simulink model "Potentiometer_Calibration"  (R2025a)
settings: Solver=ode4  StartTime=0.0  StopTime=inf  FixedStep=0.004  RelTol=1e-3  EnableMultiTasking=on
libraries: raspberrypiCommlib x2
settings Model: SimulationMode=external  ExtModeTrigDuration=2  Creator=Mustafa  LastModifiedBy=chenyihong
settings SolverCC: ExtrapolationOrder=2.0  AlgebraicLoopSolver=TrustRegion  PositivePriorityOrder=on  AutoInsertRateTranBlk=on
settings DataIOCC: ReturnWorkspaceOutputs=off
settings OptimizationCC: PassReuseOutputArgsAs=Individual arguments  MaxStackSize=200000  EfficientTunableParamExpr=on
settings DebuggingCC: ParameterTunabilityLossMsg=error  UnconnectedInputMsg=warning  UnconnectedOutputMsg=warning  UnconnectedLineMsg=warning  ArithmeticOperatorsInVariantConditions=warning
settings HardwareCC: ProdBitPerLong=64.0  ProdLargestAtomicInteger=LongLong  ProdLargestAtomicFloat=Double  ProdLongLongMode=on  ProdHWDeviceType=ARM Compatible->ARM Cortex-A (64-bit)
settings ModelReferenceCC: EnableRefExpFcnMdlSchedulingChecks=on
settings SFSimCC: SimUseLocalCustomCode=off  CustomCodeUndefinedFunction=UseInterfaceOnly
settings RTWCC: SystemTargetFile=ert.tlc  HardwareBoard=Raspberry Pi (64bit)  TLCOptions="-aInlineSetEventsForThisBaseRateFcn=TLC_FALSE -aSuppressMultiTaskScheduler=TLC_FALSE  -aRateBasedStepFcn=0"  TemplateMakefile=ert_default_tmf  GenerateReport=on  RTWUseLocalCustomCode=off  Toolchain=GNU GCC Embedded Linux  BuildConfiguration=Faster Runs  IncludeHyperlinkInReport=on  LaunchReport=on  GenerateTraceInfo=on  GenerateTraceReport=on  GenerateTraceReportSl=on  GenerateTraceReportSf=on  GenerateTraceReportEml=on  GPUComputeCapability=3.5  DLArmComputeVersion=19.05  Description=Embedded Coder
settings CodeAppCC: ForceParamTrailComments=on  IgnoreCustomStorageClasses=off  OperatorAnnotations=on  SimulinkDataObjDesc=on  SFDataObjDesc=on  InsertBlockDesc=on
settings ERTTargetCC: ExtMode=on  ExtModeTransport=2.0  ExtModeMexArgs='127.0.0.1' 0 17725  InlinedParameterPlacement=Hierarchical  DynamicArrayContainerType=coder::array  CodeReplacementLibrary=ARM Cortex-A CMSIS  SupportContinuousTime=on  SupportVariableSizeSignals=on

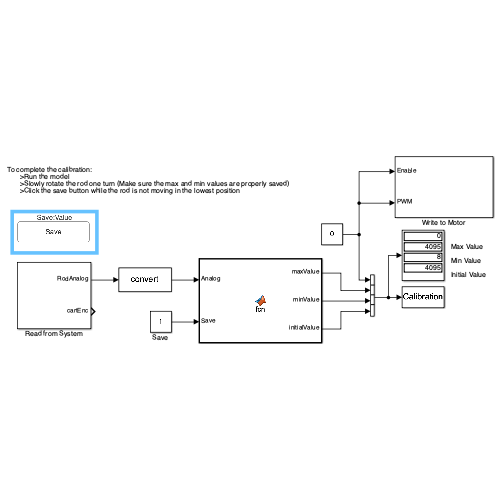
[thumbnail: Simulink's stored preview of the top-level diagram]
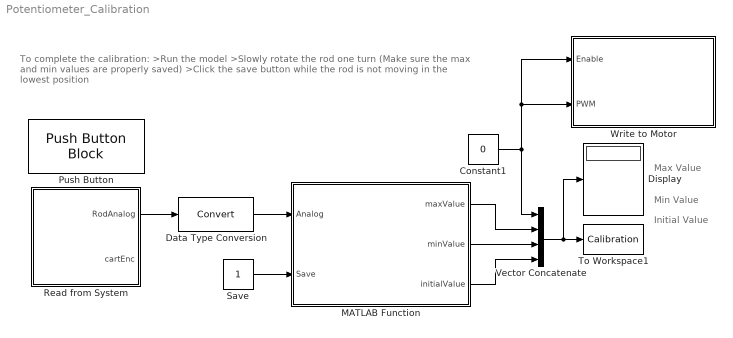
== system Potentiometer_Calibration ==
  note: Min Value
  note: To complete the calibration:
      | >Run the model
      | >Slowly rotate the rod one turn (Make sure the max and min values are properly saved)
      | >Click the save button while the rod is not moving in the lowest position
  note: Initial Value
  note: Max Value
  Constant1 : Constant  Value=0
  Data Type Conversion : DataTypeConversion  SaturateOnIntegerOverflow=off  RndMeth=Floor
  Display : Display
  MATLAB Function : MATLAB Function  TreatAsAtomicUnit=on
  Push Button : PushButtonBlock  LabelPosition=Top  ButtonText=Save  IconOnColor=[0.0, 0.39215686274509803, 0.0]  IconOffColor=[0.0, 1.0, 0.0]  OffValue=1.000000
  Read from System : Subsystem
  Save : Constant
  To Workspace1 : ToWorkspace  VariableName=Calibration  SampleTime=-1
      settings: MaxDataPoints=1
  Vector Concatenate : Concatenate  NumInputs=4
  Write to Motor : Subsystem
  wires:
  MATLAB Function/2(minValue) -> Vector Concatenate/3
  Vector Concatenate/1 -> Display/1, To Workspace1/1
  Constant1/1 -> Vector Concatenate/1, Write to Motor/2(PWM), Write to Motor/1(Enable)
  Save/1 -> MATLAB Function/2(Save)
  Data Type Conversion/1 -> MATLAB Function/1(Analog)
  Read from System/1(RodAnalog) -> Data Type Conversion/1
  MATLAB Function/1(maxValue) -> Vector Concatenate/2
  MATLAB Function/3(initialValue) -> Vector Concatenate/4

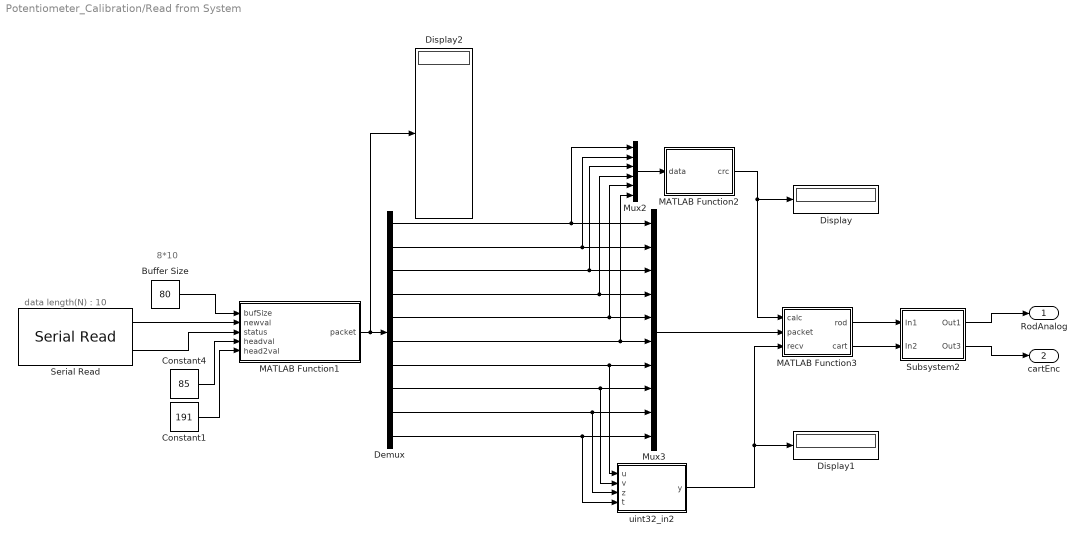
== system Potentiometer_Calibration/Read from System ==
  note: data length(N) : 10
  note: 8*10
  Buffer Size : Constant  Value=80  OutDataTypeStr=uint8
  Constant1 : Constant  Value=191  OutDataTypeStr=uint8
  Constant4 : Constant  Value=85  OutDataTypeStr=uint8
  Demux : Demux  Outputs=10
  Display : Display
  Display1 : Display
  Display2 : Display
  MATLAB Function1 : MATLAB Function  TreatAsAtomicUnit=on
  MATLAB Function2 : MATLAB Function  TreatAsAtomicUnit=on
  MATLAB Function3 : MATLAB Function  TreatAsAtomicUnit=on
  Mux2 : Mux  Inputs=6
  Mux3 : Mux  Inputs=10
  Serial Read : raspberrypiCommlib/Serial Read  board=Pi 3 Model B  SCIModule_=/dev/serial0  Baudrate_=115200  Parity=None  StopBits_=1  HardwareFlowControl=None  ByteOrder=LittleEndian  DataLength=10  DataType=uint8  OutputStatus=on  SampleTime=0.004  blockPlatform=RaspberryPi
  Subsystem2 : Subsystem
  uint32_in2 : MATLAB Function  TreatAsAtomicUnit=on
  RodAnalog : Outport
  cartEnc : Outport  Port=2
  wires:
  Subsystem2/1(Out1) -> RodAnalog/1
  MATLAB Function3/2(cart) -> Subsystem2/2(In2)
  MATLAB Function3/1(rod) -> Subsystem2/1(In1)
  Subsystem2/2(Out3) -> cartEnc/1
  Demux/7 -> Mux3/7, uint32_in2/1(u)
  MATLAB Function1/1(packet) -> Display2/1, Demux/1
  Serial Read/1 -> MATLAB Function1/2(newval)
  Constant4/1 -> MATLAB Function1/4(headval)
  Demux/5 -> Mux3/5, Mux2/5
  Demux/2 -> Mux3/2, Mux2/2
  Buffer Size/1 -> MATLAB Function1/1(bufSize)
  Mux3/1 -> MATLAB Function3/2(packet)
  Serial Read/2 -> MATLAB Function1/3(status)
  uint32_in2/1(y) -> Display1/1, MATLAB Function3/3(recv)
  MATLAB Function2/1(crc) -> Display/1, MATLAB Function3/1(calc)
  Demux/3 -> Mux3/3, Mux2/3
  Demux/9 -> Mux3/9, uint32_in2/3(z)
  Demux/4 -> Mux3/4, Mux2/4
  Demux/8 -> Mux3/8, uint32_in2/2(v)
  Demux/10 -> Mux3/10, uint32_in2/4(t)
  Constant1/1 -> MATLAB Function1/5(head2val)
  Demux/6 -> Mux3/6, Mux2/6
  Mux2/1 -> MATLAB Function2/1(data)
  Demux/1 -> Mux3/1, Mux2/1

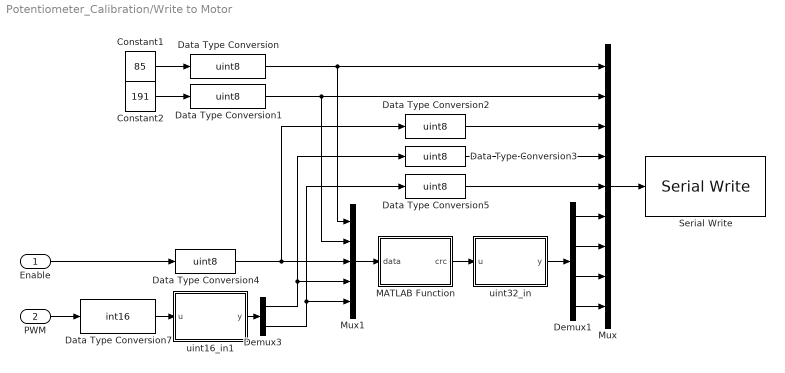
== system Potentiometer_Calibration/Write to Motor ==
  Enable : Inport
  PWM : Inport  Port=2
  Constant1 : Constant  Value=85
  Constant2 : Constant  Value=191
  Data Type Conversion{,1..5} (6 alike) : DataTypeConversion  OutDataTypeStr=uint8  SaturateOnIntegerOverflow=off  RndMeth=Floor
  Data Type Conversion7 : DataTypeConversion  OutDataTypeStr=int16  SaturateOnIntegerOverflow=off  RndMeth=Floor
  Demux1 : Demux
  Demux3 : Demux  Outputs=2
  MATLAB Function : MATLAB Function  TreatAsAtomicUnit=on
  Mux : Mux  Inputs=9
  Mux1 : Mux  Inputs=5
  Serial Write : raspberrypiCommlib/Serial Write  board=Pi 3 Model B  SCIModule_=/dev/serial0  Baudrate_=115200  Parity=None  StopBits_=1  HardwareFlowControl=None  ByteOrder=LittleEndian  OutputStatus=off  blockPlatform=RaspberryPi
  uint16_in1 : MATLAB Function  TreatAsAtomicUnit=on
  uint32_in : MATLAB Function  TreatAsAtomicUnit=on
  wires:
  Data Type Conversion7/1 -> uint16_in1/1(u)
  uint16_in1/1(y) -> Demux3/1
  Data Type Conversion5/1 -> Mux/5
  Demux3/1 -> Data Type Conversion3/1, Mux1/4
  Data Type Conversion/1 -> Mux/1, Mux1/1
  Data Type Conversion3/1 -> Mux/4
  Data Type Conversion1/1 -> Mux/2, Mux1/2
  Mux/1 -> Serial Write/1
  Data Type Conversion2/1 -> Mux/3
  uint32_in/1(y) -> Demux1/1
  MATLAB Function/1(crc) -> uint32_in/1(u)
  Mux1/1 -> MATLAB Function/1(data)
  Constant2/1 -> Data Type Conversion1/1
  Constant1/1 -> Data Type Conversion/1
  PWM/1 -> Data Type Conversion7/1
  Demux3/2 -> Data Type Conversion5/1, Mux1/5
  Demux1/4 -> Mux/9
  Demux1/3 -> Mux/8
  Demux1/2 -> Mux/7
  Demux1/1 -> Mux/6
  Data Type Conversion4/1 -> Mux1/3, Data Type Conversion2/1
  Enable/1 -> Data Type Conversion4/1

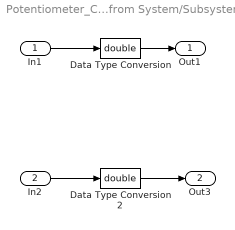
== system Potentiometer_Calibration/Read from System/Subsystem2 ==
  In1 : Inport
  In2 : Inport  Port=2
  Data Type Conversion : DataTypeConversion  OutDataTypeStr=double  SaturateOnIntegerOverflow=off  RndMeth=Floor
  Data Type Conversion2 : DataTypeConversion  OutDataTypeStr=double  SaturateOnIntegerOverflow=off  RndMeth=Floor
  Out1 : Outport
  Out3 : Outport  Port=2
  wires:
  Data Type Conversion2/1 -> Out3/1
  Data Type Conversion/1 -> Out1/1
  In2/1 -> Data Type Conversion2/1
  In1/1 -> Data Type Conversion/1

== matlab function Potentiometer_Calibration/MATLAB Function ==
  data: Analog input; maxValue output; Save input; minValue output; initialValue output
function [maxValue,minValue,initialValue] = fcn(Analog,Save)
    persistent maxAnalog
    if isempty(maxAnalog)
        maxAnalog=500;
    end
    persistent minAnalog
    if isempty(minAnalog)
        minAnalog=500;
    end
    if (Analog>maxAnalog)
        maxAnalog=Analog;
    end
    if (minAnalog > Analog)
        if (Analog  ~= 0)
            minAnalog=Analog;
        end
    end
    if (Save==1)
        maxValue=maxAnalog;
        minValue=minAnalog;
        initialValue=Analog;
    else
        maxValue=500;
        minValue=500;
        initialValue=Analog;
    end
end

== matlab function Potentiometer_Calibration/Write to Motor/MATLAB Function ==
  data: data input; crc output
function crc = crc_32(data)

% Computes the CRC-32/MPEG-2 checksum value of a byte vector.
% Uses a left shifting (not reflected) CRC along with the 
% CRC polynomial 0x04C11DB7 and initial CRC value of 0xFFFFFFFF,
% and is not post complemented.
%--------------------------------------------------------------------------
%   Version:    130
%   Programmer: Oliver Calderbank
%   Date:       21-07-2019

% Initialize variables
crc  = uint32(hex2dec('FFFFFFFF'));
poly = uint32(hex2dec('04C11DB7'));
data = uint8(data);
temp = uint32(data);

for i = 1:length(data)
    % xor next byte to upper bits of crc
    crc = bitxor(crc,uint32(bitshift(temp(i),24)));
    for j = 1:8
        msb = bitsra(crc,31);
        crc = bitsll(crc,1);
        if msb == 1 
            crc = bitxor(crc,poly);
        end 
    end
end
end

== matlab function Potentiometer_Calibration/Write to Motor/uint16_in1 ==
  data: u input; y output
function y = fcn(u)
t=typecast(int16(u),'uint8');
y = [t(1) t(2)];

== matlab function Potentiometer_Calibration/Write to Motor/uint32_in ==
  data: u input; y output
function y = fcn(u)
t=typecast(uint32(u),'uint8');
y = [t(1) t(2) t(3) t(4)];

== matlab function Potentiometer_Calibration/Read from System/MATLAB Function1 ==
  settings: updateMethod=DISCRETE
  data: bufSize input uint8 size=1; newval input uint8 size=10; status input; headval input uint8; packet output size=10; head2val input
function packet   = fcn(bufSize,newval,status,headval,head2val)
%initializing
persistent val;
persistent bff;
persistent packetindex
if isempty(bff)
    packetindex =uint8(zeros(1,10));
end
if isempty(val)
    val=0;
    bff = zeros(bufSize,1); %initializing
    inc=0;
else
    inc=1;
end

ind =uint8( mod(val-1,bufSize) + 1); %current index
if isempty(bff)
    bff = zeros(bufSize,1); %initializing
end
if status==0  %UART Status
    for i = 1:1:10
        bff(mod(ind-1+i-1,bufSize)+1) = newval(i); %adding the circular buffer
    end
    if inc==1
        val=val+10;   
    end
end
if ind==0
    val=0;
end
buffout =uint8( bff((1:80)));  % whole buffer
head=uint8(find(bff(ind+1:end)==headval)+double(ind)); %finding first header
if isempty(head)
    head=uint8(find(bff(1:end)==headval));
end
if bff(mod(head(1),bufSize)+1)==head2val %header2 check
    packetindex=[mod(head(1)-1,bufSize)+1 mod(head(1),bufSize)+1 mod(head(1)+1,bufSize)+1 mod(head(1)+2,bufSize)+1 ... %adding correct package's index to array
                 mod(head(1)+3,bufSize)+1 mod(head(1)+4,bufSize)+1 mod(head(1)+5,bufSize)+1 mod(head(1)+6,bufSize)+1 mod(head(1)+7,bufSize)+1 mod(head(1)+8,bufSize)+1];
end
lastadd=uint8(bff(head(1)+1));
packet=bff(packetindex);

== matlab function Potentiometer_Calibration/Read from System/MATLAB Function2 ==
  data: data input; crc output
function crc = crc_32(data)

% Computes the CRC-32/MPEG-2 checksum value of a byte vector.
% Uses a left shifting (not reflected) CRC along with the 
% CRC polynomial 0x04C11DB7 and initial CRC value of 0xFFFFFFFF,
% and is not post complemented.
%--------------------------------------------------------------------------
%   Version:    130
%   Programmer: Oliver Calderbank
%   Date:       21-07-2019

% Initialize variables
crc  = uint32(hex2dec('FFFFFFFF'));
poly = uint32(hex2dec('04C11DB7'));
data = uint8(data);
temp = uint32(data);

for i = 1:length(data)
    % xor next byte to upper bits of crc
    crc = bitxor(crc,uint32(bitshift(temp(i),24)));
    for j = 1:8
        msb = bitsra(crc,31);
        crc = bitsll(crc,1);
        if msb == 1 
            crc = bitxor(crc,poly);
        end 
    end
end
end

== matlab function Potentiometer_Calibration/Read from System/MATLAB Function3 ==
  data: calc input; packet input; rod output int16 size=1; recv input; cart output int16 size=1
function [rod,cart] = fcn(calc,packet,recv)
persistent validpack;
persistent validpack2;
if isempty(validpack)
    Axisx=[packet(3) packet(4)];
    validpack=typecast(uint8(Axisx),'int16');
end
if isempty(validpack2)
    Axisy=[packet(5) packet(6)];
    validpack2=typecast(uint8(Axisy),'int16');
end
if calc==recv
    Axisx=[packet(3) packet(4)];
    validpack=typecast(uint8(Axisx),'int16');
    Axisy=[packet(5) packet(6)];
    validpack2=typecast(uint8(Axisy),'int16');
    rod=validpack;
    cart=validpack2;
else
	rod=validpack;
    cart=validpack2;
end

== matlab function Potentiometer_Calibration/Read from System/uint32_in2 ==
  data: u input; y output uint32 size=1; v input; z input; t input
function y = fcn(u,v,z,t)
x=[u v z t];
k=typecast(uint8(x),'uint32');
y = k;
